simulink model "quadSimplifiedModel"  (R2018b)
settings: Solver=FixedStepAuto  StartTime=0.0  StopTime=tfinal  FixedStep=dt  RelTol=1e-3
values from neighbouring files (symbols this model uses):
  dt = 0.005    [quadSimRunMain.m]    (also in runquadXModel.m)
  Gain = [1 0, 0 0,0 0, 0 0;     0 1, 0 0, 0 0, 0 0;     0 0, param.dt 0, 0 0, 0 0;     0 0, 0 param.dt, 0 0, 0 0;     0 0, 0 0, param.dt^2/2 0, 0 0;     0 0, 0 0, 0 param.dt^2/2, 0 0;     0 0, 0 0, 0 0, 1 0;     0 0, 0 0, 0 0, 0 1]    [quadSimRunMain.m]
  Kdphi = 0.0478*1    (= 0.0478)    [quadSimRunMain.m]
  Kdpsi = 0.067644*1    (= 0.067644)    [quadSimRunMain.m]
  Kdtheta = 0.0478*1    (= 0.0478)    [quadSimRunMain.m]
  Kdx = 15    [quadSimRunMain.m]
  Kdy = 15    [quadSimRunMain.m]
  Kdz = 5.5    [quadSimRunMain.m]
  Kiphi = 0.0098*0    (= 0)    [quadSimRunMain.m]
  Kipsi = 0.045028*.0    (= 0)    [quadSimRunMain.m]
  Kitheta = 0.0098*0    (= 0)    [quadSimRunMain.m]
  Kix = 1    [quadSimRunMain.m]
  Kiy = 1    [quadSimRunMain.m]
  Kiz = 1.5    [quadSimRunMain.m]
  Kpphi = 0.0439*1    (= 0.0439)    [quadSimRunMain.m]
  Kppsi = 0.11038*1    (= 0.11038)    [quadSimRunMain.m]
  Kptheta = 0.0439*1    (= 0.0439)    [quadSimRunMain.m]
  Kpx = 5    [quadSimRunMain.m]
  Kpy = 5    [quadSimRunMain.m]
  Kpz = 3.5    [quadSimRunMain.m]
  Nphi = 1/Tfphi    (= 162.638649449)    [quadSimRunMain.m]
  Npsi = 1/Tfpsi    (= 159.182438993)    [quadSimRunMain.m]
  Ntheta = 1/Tftheta    (= 162.638649449)    [quadSimRunMain.m]
  Nx = 1/0.002099    (= 476.417341591)    [quadSimRunMain.m]
  Ny = 1/0.002099    (= 476.417341591)    [quadSimRunMain.m]
  Nz = 1/0.002099    (= 476.417341591)    [quadSimRunMain.m]
  pathSelect = 1    [quadSimRunMain.m]
  Uphisat = 100*param.m*param.g(3)*0.5    [quadSimRunMain.m]
  Upsisat = 100*param.m*param.g(3)*0.1    [quadSimRunMain.m]
  Uthetasat = 100*param.m*param.g(3)*0.5    [quadSimRunMain.m]
  Uzsat = 100*3*param.m*param.g(3)    [quadSimRunMain.m]
undefined symbols (not defined in the file or in its folder): sigbuilder_block, sigeul, sigpos
libraries: simulink x12
settings Model: Creator=duho46  LastModifiedBy=duho46

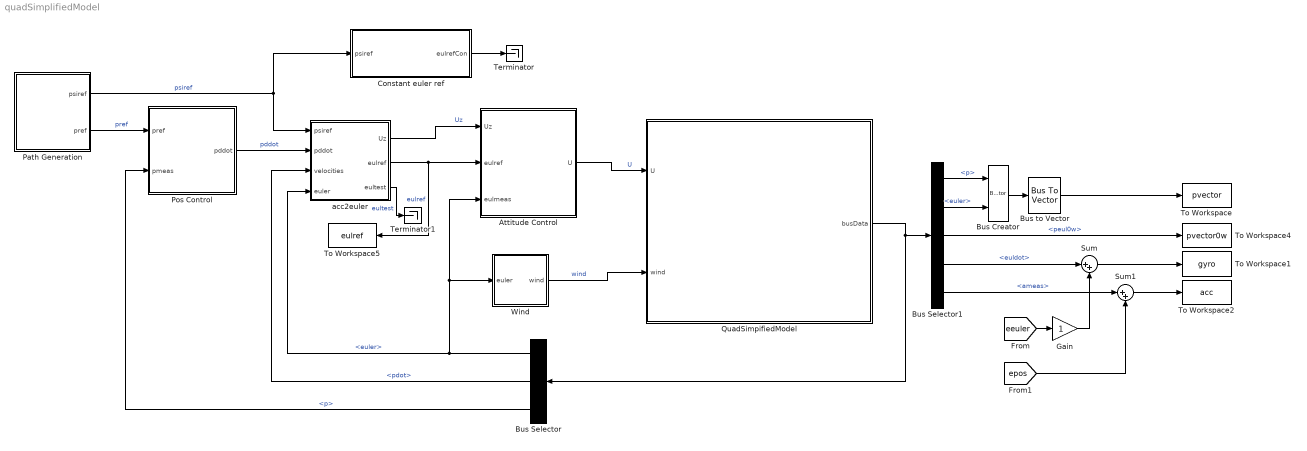
== system quadSimplifiedModel ==
  Attitude Control : Subsystem
      mask Display: image('C:\Users\duho46\Pictures\angles.png');
  Bus Creator : BusCreator  Inputs=2
  Bus Selector : BusSelector  OutputSignals=euler,pdot,p
  Bus Selector1 : BusSelector  OutputSignals=p,euler,peul0w,euldot,ameas
  Bus to Vector : BusToVector
  "Constant euler ref " : Subsystem
  Gain : Gain
  Path Generation : Subsystem
      mask Display: image('C:\Users\duho46\Pictures\96643.png');
  Pos Control : Subsystem
      mask Display: image('C:\Users\duho46\Pictures\control.png');
  QuadSimpifiedModel : Subsystem
      mask Display: image('C:\Users\duho46\Pictures\DJI Mavic Pro.jpg');
  Sum : Sum  Inputs=|++
  Sum1 : Sum  Inputs=|++
  Terminator : Terminator
  Terminator1 : Terminator
  To Workspace : ToWorkspace  VariableName=pvector  SampleTime=-1
  To Workspace1 : ToWorkspace  VariableName=gyro  SampleTime=-1
  To Workspace2 : ToWorkspace  VariableName=acc  SampleTime=-1
  To Workspace4 : ToWorkspace  VariableName=pvector0w  SampleTime=-1
  To Workspace5 : ToWorkspace  VariableName=eulref  SampleTime=-1
  Wind : Subsystem
      mask Display: image('C:\Users\duho46\Pictures\wind.png');
  acc2euler : MATLAB Function  TreatAsAtomicUnit=on
  wires:
  Path Generation/2(pref) -> Pos Control/1(pref)  "pref"
  Pos Control/1(pddot) -> acc2euler/2(pddot)  "pddot"
  acc2euler/1(Uz) -> Attitude Control/1(Uz)  "Uz"
  acc2euler/2(eulref) -> To Workspace5/1, Attitude Control/2(eulref)  "eulref"
  Attitude Control/1(U) -> QuadSimpifiedModel/1(U)  "U"
  Wind/1(wind) -> QuadSimpifiedModel/2(wind)  "wind"
  QuadSimpifiedModel/1(busData) -> Bus Selector/1, Bus Selector1/1
  Bus Selector/1 -> acc2euler/4(euler), Wind/1(euler), Attitude Control/3(eulmeas)  "<euler>"
  Bus Selector/2 -> acc2euler/3(velocities)  "<pdot>"
  Bus Selector/3 -> Pos Control/2(pmeas)  "<p>"
  Bus Selector1/3 -> To Workspace4/1  "<peul0w>"
  Bus to Vector/1 -> To Workspace/1
  Bus Selector1/1 -> Bus Creator/1  "<p>"
  Bus Selector1/2 -> Bus Creator/2  "<euler>"
  Bus Creator/1 -> Bus to Vector/1
  Bus Selector1/4 -> Sum/1  "<euldot>"
  Sum/1 -> To Workspace1/1
  Bus Selector1/5 -> Sum1/1  "<ameas>"
  Sum1/1 -> To Workspace2/1
  [eeuler] -> Gain/1
  [epos] -> Sum1/2
  Gain/1 -> Sum/2
  Path Generation/1(psiref) -> "Constant euler ref "/1(psiref), acc2euler/1(psiref)  "psiref"
  "Constant euler ref "/1(eulrefCon) -> Terminator/1
  acc2euler/3(eultest) -> Terminator1/1  "eultest"

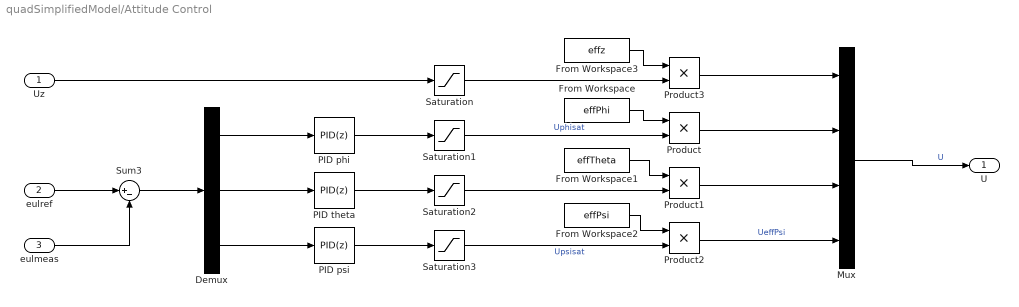
== system quadSimplifiedModel/Attitude Control ==
  Uz : Inport
  eulref : Inport  Port=2
  eulmeas : Inport  Port=3
  Demux : Demux  Outputs=3
  From Workspace : FromWorkspace  VariableName=effPhi  SampleTime=0
  From Workspace1 : FromWorkspace  VariableName=effTheta  SampleTime=0
  From Workspace2 : FromWorkspace  VariableName=effPsi  SampleTime=0
  From Workspace3 : FromWorkspace  VariableName=effz  SampleTime=0
  Mux : Mux
  PID phi : simulink/Continuous/PID Controller  Controller=PID  Form=Parallel  TimeDomain=Discrete-time  SampleTime=-1  IntegratorMethod=Forward Euler  FilterMethod=Forward Euler  ControllerParametersSource=internal  P=Kpphi  I=Kiphi  D=Kdphi  UseFilter=off  N=Nphi  TunerSelectOption=Transfer Function Based (PID Tuner App)  InitialConditionSource=internal  InitialConditionForIntegrator=0  InitialConditionForFilter=0  DifferentiatorICPrevScaledInput=0  ExternalReset=none  TrackingMode=off  Kt=1  LimitOutput=off  UpperSaturationLimit=inf  LowerSaturationLimit=-inf  LinearizeAsGain=on  AntiWindupMode=none  Kb=1  POutMin=[]  POutMax=[]  IOutMin=[]  IOutMax=[]  DOutMin=[]  DOutMax=[]  NOutMin=[]  NOutMax=[]  SumOutMin=[]  SumOutMax=[]  SaturationOutMin=[]  SaturationOutMax=[]  PParamMin=[]  PParamMax=[]  IParamMin=[]  IParamMax=[]  DParamMin=[]  DParamMax=[]  NParamMin=[]  NParamMax=[]  KbParamMin=[]  KbParamMax=[]  KtParamMin=[]  KtParamMax=[]  KbOutMin=[]  KbOutMax=[]  KtOutMin=[]  KtOutMax=[]  IntegratorOutMin=[]  IntegratorOutMax=[]  FilterOutMin=[]  FilterOutMax=[]  SumI1OutMin=[]  SumI1OutMax=[]  SumI2OutMin=[]  SumI2OutMax=[]  SumI3OutMin=[]  SumI3OutMax=[]  SumI4OutMin=[]  SumI4OutMax=[]  SumDOutMin=[]  SumDOutMax=[]  DifferentiatorOutMin=[]  DifferentiatorOutMax=[]  FilterDiffOutCoefMin=[]  FilterDiffOutCoefMax=[]  ReciprocalOutMin=[]  ReciprocalOutMax=[]  SumDenOutMin=[]  SumDenOutMax=[]  SumNumOutMin=[]  SumNumOutMax=[]  DivideOutMin=[]  DivideOutMax=[]  IntegratorContinuousStateAttributes=''  IntegratorStateMustResolveToSignalObject=off  IntegratorRTWStateStorageClass=Auto  FilterContinuousStateAttributes=''  FilterStateMustResolveToSignalObject=off  FilterRTWStateStorageClass=Auto  ParallelPVariant=InternalParameters  IdealPVariant=Disabled  IVariant=InternalParameters  DVariant=InternalParameters  IntegratorVariant=Discrete  SatVariant=Disabled  AWVariant=Passthrough  PCopyVariant=Disabled  TRVariant=Disabled  FdbkBlocksVariant=Forward  IdealPFdbkVariant=Disabled  SatFdbkVariant=Disabled  DerivativeFilterVariant=Differentiator  NVariant=Passthrough  NCopyVariant=Disabled_SignalSpec  FilterICVariant=InternalICsDifferentiator  IntegratorICVariant=InternalICs  ExternalResetVariant=Disabled  TRSumVariant=Passthrough  SumFdbkVariant=Disabled  SumVariant=Sum_PID
  PID psi : simulink/Continuous/PID Controller  Controller=PID  Form=Parallel  TimeDomain=Discrete-time  SampleTime=-1  IntegratorMethod=Forward Euler  FilterMethod=Forward Euler  ControllerParametersSource=internal  P=Kppsi  I=Kipsi  D=Kdpsi  UseFilter=off  N=Npsi  TunerSelectOption=Transfer Function Based (PID Tuner App)  InitialConditionSource=internal  InitialConditionForIntegrator=0  InitialConditionForFilter=0  DifferentiatorICPrevScaledInput=0  ExternalReset=none  TrackingMode=off  Kt=1  LimitOutput=off  UpperSaturationLimit=inf  LowerSaturationLimit=-inf  LinearizeAsGain=on  AntiWindupMode=none  Kb=1  POutMin=[]  POutMax=[]  IOutMin=[]  IOutMax=[]  DOutMin=[]  DOutMax=[]  NOutMin=[]  NOutMax=[]  SumOutMin=[]  SumOutMax=[]  SaturationOutMin=[]  SaturationOutMax=[]  PParamMin=[]  PParamMax=[]  IParamMin=[]  IParamMax=[]  DParamMin=[]  DParamMax=[]  NParamMin=[]  NParamMax=[]  KbParamMin=[]  KbParamMax=[]  KtParamMin=[]  KtParamMax=[]  KbOutMin=[]  KbOutMax=[]  KtOutMin=[]  KtOutMax=[]  IntegratorOutMin=[]  IntegratorOutMax=[]  FilterOutMin=[]  FilterOutMax=[]  SumI1OutMin=[]  SumI1OutMax=[]  SumI2OutMin=[]  SumI2OutMax=[]  SumI3OutMin=[]  SumI3OutMax=[]  SumI4OutMin=[]  SumI4OutMax=[]  SumDOutMin=[]  SumDOutMax=[]  DifferentiatorOutMin=[]  DifferentiatorOutMax=[]  FilterDiffOutCoefMin=[]  FilterDiffOutCoefMax=[]  ReciprocalOutMin=[]  ReciprocalOutMax=[]  SumDenOutMin=[]  SumDenOutMax=[]  SumNumOutMin=[]  SumNumOutMax=[]  DivideOutMin=[]  DivideOutMax=[]  IntegratorContinuousStateAttributes=''  IntegratorStateMustResolveToSignalObject=off  IntegratorRTWStateStorageClass=Auto  FilterContinuousStateAttributes=''  FilterStateMustResolveToSignalObject=off  FilterRTWStateStorageClass=Auto  ParallelPVariant=InternalParameters  IdealPVariant=Disabled  IVariant=InternalParameters  DVariant=InternalParameters  IntegratorVariant=Discrete  SatVariant=Disabled  AWVariant=Passthrough  PCopyVariant=Disabled  TRVariant=Disabled  FdbkBlocksVariant=Forward  IdealPFdbkVariant=Disabled  SatFdbkVariant=Disabled  DerivativeFilterVariant=Differentiator  NVariant=Passthrough  NCopyVariant=Disabled_SignalSpec  FilterICVariant=InternalICsDifferentiator  IntegratorICVariant=InternalICs  ExternalResetVariant=Disabled  TRSumVariant=Passthrough  SumFdbkVariant=Disabled  SumVariant=Sum_PID
  PID theta : simulink/Continuous/PID Controller  Controller=PID  Form=Parallel  TimeDomain=Discrete-time  SampleTime=-1  IntegratorMethod=Forward Euler  FilterMethod=Forward Euler  ControllerParametersSource=internal  P=Kptheta  I=Kitheta  D=Kdtheta  UseFilter=off  N=Ntheta  TunerSelectOption=Transfer Function Based (PID Tuner App)  InitialConditionSource=internal  InitialConditionForIntegrator=0  InitialConditionForFilter=0  DifferentiatorICPrevScaledInput=0  ExternalReset=none  TrackingMode=off  Kt=1  LimitOutput=off  UpperSaturationLimit=inf  LowerSaturationLimit=-inf  LinearizeAsGain=on  AntiWindupMode=none  Kb=1  POutMin=[]  POutMax=[]  IOutMin=[]  IOutMax=[]  DOutMin=[]  DOutMax=[]  NOutMin=[]  NOutMax=[]  SumOutMin=[]  SumOutMax=[]  SaturationOutMin=[]  SaturationOutMax=[]  PParamMin=[]  PParamMax=[]  IParamMin=[]  IParamMax=[]  DParamMin=[]  DParamMax=[]  NParamMin=[]  NParamMax=[]  KbParamMin=[]  KbParamMax=[]  KtParamMin=[]  KtParamMax=[]  KbOutMin=[]  KbOutMax=[]  KtOutMin=[]  KtOutMax=[]  IntegratorOutMin=[]  IntegratorOutMax=[]  FilterOutMin=[]  FilterOutMax=[]  SumI1OutMin=[]  SumI1OutMax=[]  SumI2OutMin=[]  SumI2OutMax=[]  SumI3OutMin=[]  SumI3OutMax=[]  SumI4OutMin=[]  SumI4OutMax=[]  SumDOutMin=[]  SumDOutMax=[]  DifferentiatorOutMin=[]  DifferentiatorOutMax=[]  FilterDiffOutCoefMin=[]  FilterDiffOutCoefMax=[]  ReciprocalOutMin=[]  ReciprocalOutMax=[]  SumDenOutMin=[]  SumDenOutMax=[]  SumNumOutMin=[]  SumNumOutMax=[]  DivideOutMin=[]  DivideOutMax=[]  IntegratorContinuousStateAttributes=''  IntegratorStateMustResolveToSignalObject=off  IntegratorRTWStateStorageClass=Auto  FilterContinuousStateAttributes=''  FilterStateMustResolveToSignalObject=off  FilterRTWStateStorageClass=Auto  ParallelPVariant=InternalParameters  IdealPVariant=Disabled  IVariant=InternalParameters  DVariant=InternalParameters  IntegratorVariant=Discrete  SatVariant=Disabled  AWVariant=Passthrough  PCopyVariant=Disabled  TRVariant=Disabled  FdbkBlocksVariant=Forward  IdealPFdbkVariant=Disabled  SatFdbkVariant=Disabled  DerivativeFilterVariant=Differentiator  NVariant=Passthrough  NCopyVariant=Disabled_SignalSpec  FilterICVariant=InternalICsDifferentiator  IntegratorICVariant=InternalICs  ExternalResetVariant=Disabled  TRSumVariant=Passthrough  SumFdbkVariant=Disabled  SumVariant=Sum_PID
  Product{,1..3} (4 alike) : Product
  Saturation : Saturate  UpperLimit=Uzsat  LowerLimit=-Uzsat
  Saturation1 : Saturate  UpperLimit=Uphisat  LowerLimit=-Uphisat
  Saturation2 : Saturate  UpperLimit=Uthetasat  LowerLimit=-Uthetasat
  Saturation3 : Saturate  UpperLimit=Upsisat  LowerLimit=-Upsisat
  Sum3 : Sum  Inputs=|+-
  U : Outport
  wires:
  PID phi/1 -> Saturation1/1
  Mux/1 -> U/1  "U"
  Demux/3 -> PID psi/1
  PID theta/1 -> Saturation2/1
  PID psi/1 -> Saturation3/1
  Demux/2 -> PID theta/1
  Uz/1 -> Saturation/1
  Sum3/1 -> Demux/1
  eulref/1 -> Sum3/1
  eulmeas/1 -> Sum3/2
  Demux/1 -> PID phi/1
  Saturation1/1 -> Product/2  "Uphisat"
  From Workspace/1 -> Product/1
  Product/1 -> Mux/2
  Product1/1 -> Mux/3
  Product2/1 -> Mux/4  "UeffPsi"
  Saturation3/1 -> Product2/2  "Upsisat"
  Saturation2/1 -> Product1/2
  From Workspace1/1 -> Product1/1
  From Workspace2/1 -> Product2/1
  Product3/1 -> Mux/1
  Saturation/1 -> Product3/2
  From Workspace3/1 -> Product3/1

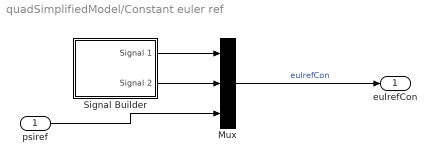
== system quadSimplifiedModel/Constant euler ref  ==
  psiref : Inport
  Mux : Mux  Inputs=3
  Signal Builder : Subsystem  Tag=STV Subsys  LoadFcn=sigbuilder_block('load');  StartFcn=sigbuilder_block('start');  StopFcn=sigbuilder_block('stop');  ClipboardFcn=sigbuilder_block('clipboard');  mask(Sigbuilder block){tuvar=[0:10]}
      mask help: Simulink:masks:SigbuilderBlock_MD
      mask init:
      | if ~strcmp(get_param(bdroot(gcbh),'SimulationStatus'),'stopped') tuvar = sigbuilder_block('maskInit'); end
      settings: CopyFcn=sigbuilder_block('copy');  DeleteFcn=sigbuilder_block('delete');  ModelCloseFcn=sigbuilder_block('modelClose');  PreSaveFcn=sigbuilder_block('preSave');  PauseFcn=sigbuilder_block('pause');  ContinueFcn=sigbuilder_block('continue');  NameChangeFcn=sigbuilder_block('namechange');  OpenFcn=sigbuilder_block('open',[1692 200.25 550.5 399.75 ]);  CloseFcn=sigbuilder_block('close');
      mask Display: plot(0, 0, 100, 100,[2, 2, 32, 32, 2], [68, 8, 8, 68, 68],[32, 2], [38, 38], [32, 19, 2],[53, 60, 44], [32, 17, 17, 2],[16, 16, 31, 31]);txt = getActiveGroup(gcbh);text(2, 100, txt,'verticalAlignment', 'top');
  eulrefCon : Outport
  wires:
  Signal Builder/1(Signal 1) -> Mux/1
  psiref/1 -> Mux/3
  Mux/1 -> eulrefCon/1  "eulrefCon"
  Signal Builder/2(Signal 2) -> Mux/2

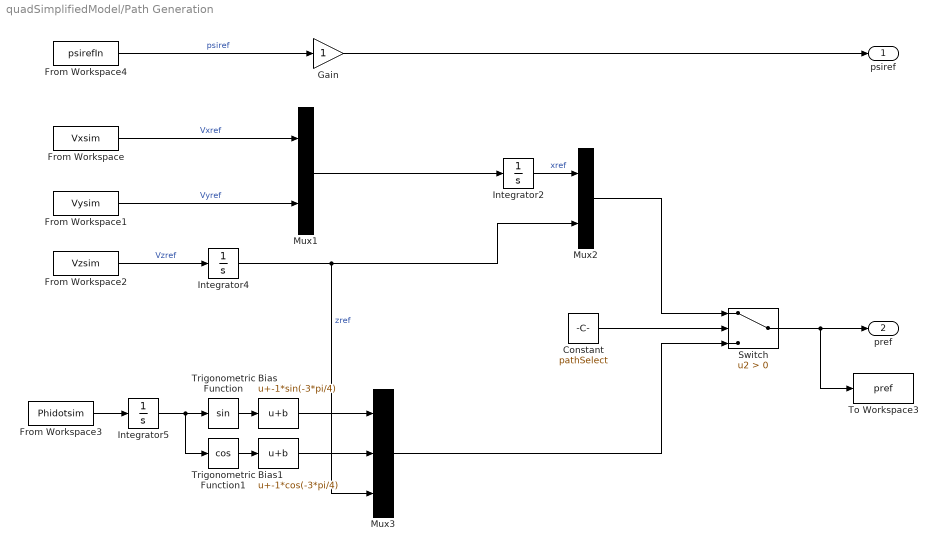
== system quadSimplifiedModel/Path Generation ==
  Bias : Bias  Bias=-1*sin(-3*pi/4)
  Bias1 : Bias  Bias=-1*cos(-3*pi/4)
  Constant : Constant  Value=pathSelect
  From Workspace : FromWorkspace  VariableName=Vxsim  SampleTime=0
  From Workspace1 : FromWorkspace  VariableName=Vysim  SampleTime=0
  From Workspace2 : FromWorkspace  VariableName=Vzsim  SampleTime=0
  From Workspace3 : FromWorkspace  VariableName=Phidotsim  SampleTime=0
  From Workspace4 : FromWorkspace  VariableName=psirefIn  SampleTime=0
  Gain : Gain
  Integrator2 : Integrator
  Integrator4 : Integrator
  Integrator5 : Integrator  InitialCondition=-3*pi/4
  Mux1 : Mux  Inputs=2
  Mux2 : Mux  Inputs=2
  Mux3 : Mux  Inputs=3
  Switch : Switch  Criteria=u2 > Threshold
  To Workspace3 : ToWorkspace  VariableName=pref  SampleTime=-1
  Trigonometric Function : Trigonometry
  Trigonometric Function1 : Trigonometry  Operator=cos
  psiref : Outport
  pref : Outport  Port=2
  wires:
  Integrator4/1 -> Mux3/3, Mux2/2  "zref"
  From Workspace2/1 -> Integrator4/1  "Vzref"
  Integrator5/1 -> Trigonometric Function1/1, Trigonometric Function/1
  From Workspace3/1 -> Integrator5/1
  Trigonometric Function1/1 -> Bias1/1
  Trigonometric Function/1 -> Bias/1
  Bias/1 -> Mux3/1
  Bias1/1 -> Mux3/2
  From Workspace4/1 -> Gain/1  "psiref"
  Mux1/1 -> Integrator2/1
  Integrator2/1 -> Mux2/1  "xref"
  From Workspace/1 -> Mux1/1  "Vxref"
  From Workspace1/1 -> Mux1/2  "Vyref"
  Gain/1 -> psiref/1
  Switch/1 -> To Workspace3/1, pref/1
  Mux2/1 -> Switch/1
  Mux3/1 -> Switch/3
  Constant/1 -> Switch/2

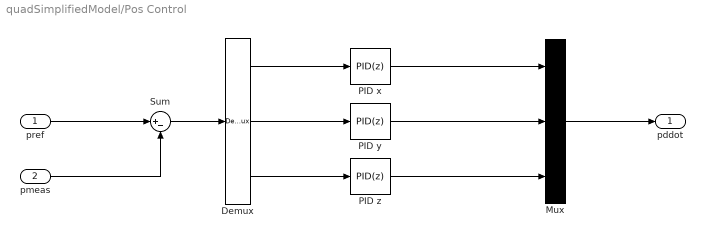
== system quadSimplifiedModel/Pos Control ==
  pref : Inport
  pmeas : Inport  Port=2
  Demux : Demux  Outputs=3
  Mux : Mux  Inputs=3
  PID x : simulink/Continuous/PID Controller  Controller=PID  Form=Parallel  TimeDomain=Discrete-time  SampleTime=-1  IntegratorMethod=Forward Euler  FilterMethod=Forward Euler  ControllerParametersSource=internal  P=Kpx  I=Kix  D=Kdx  UseFilter=off  N=Nx  TunerSelectOption=Transfer Function Based (PID Tuner App)  InitialConditionSource=internal  InitialConditionForIntegrator=0  InitialConditionForFilter=0  DifferentiatorICPrevScaledInput=0  ExternalReset=none  TrackingMode=off  Kt=1  LimitOutput=off  UpperSaturationLimit=inf  LowerSaturationLimit=-inf  LinearizeAsGain=on  AntiWindupMode=none  Kb=1  POutMin=[]  POutMax=[]  IOutMin=[]  IOutMax=[]  DOutMin=[]  DOutMax=[]  NOutMin=[]  NOutMax=[]  SumOutMin=[]  SumOutMax=[]  SaturationOutMin=[]  SaturationOutMax=[]  PParamMin=[]  PParamMax=[]  IParamMin=[]  IParamMax=[]  DParamMin=[]  DParamMax=[]  NParamMin=[]  NParamMax=[]  KbParamMin=[]  KbParamMax=[]  KtParamMin=[]  KtParamMax=[]  KbOutMin=[]  KbOutMax=[]  KtOutMin=[]  KtOutMax=[]  IntegratorOutMin=[]  IntegratorOutMax=[]  FilterOutMin=[]  FilterOutMax=[]  SumI1OutMin=[]  SumI1OutMax=[]  SumI2OutMin=[]  SumI2OutMax=[]  SumI3OutMin=[]  SumI3OutMax=[]  SumI4OutMin=[]  SumI4OutMax=[]  SumDOutMin=[]  SumDOutMax=[]  DifferentiatorOutMin=[]  DifferentiatorOutMax=[]  FilterDiffOutCoefMin=[]  FilterDiffOutCoefMax=[]  ReciprocalOutMin=[]  ReciprocalOutMax=[]  SumDenOutMin=[]  SumDenOutMax=[]  SumNumOutMin=[]  SumNumOutMax=[]  DivideOutMin=[]  DivideOutMax=[]  IntegratorContinuousStateAttributes=''  IntegratorStateMustResolveToSignalObject=off  IntegratorRTWStateStorageClass=Auto  FilterContinuousStateAttributes=''  FilterStateMustResolveToSignalObject=off  FilterRTWStateStorageClass=Auto  ParallelPVariant=InternalParameters  IdealPVariant=Disabled  IVariant=InternalParameters  DVariant=InternalParameters  IntegratorVariant=Discrete  SatVariant=Disabled  AWVariant=Passthrough  PCopyVariant=Disabled  TRVariant=Disabled  FdbkBlocksVariant=Forward  IdealPFdbkVariant=Disabled  SatFdbkVariant=Disabled  DerivativeFilterVariant=Differentiator  NVariant=Passthrough  NCopyVariant=Disabled_SignalSpec  FilterICVariant=InternalICsDifferentiator  IntegratorICVariant=InternalICs  ExternalResetVariant=Disabled  TRSumVariant=Passthrough  SumFdbkVariant=Disabled  SumVariant=Sum_PID
  PID y : simulink/Continuous/PID Controller  Controller=PID  Form=Parallel  TimeDomain=Discrete-time  SampleTime=-1  IntegratorMethod=Forward Euler  FilterMethod=Forward Euler  ControllerParametersSource=internal  P=Kpy  I=Kiy  D=Kdy  UseFilter=off  N=Ny  TunerSelectOption=Transfer Function Based (PID Tuner App)  InitialConditionSource=internal  InitialConditionForIntegrator=0  InitialConditionForFilter=0  DifferentiatorICPrevScaledInput=0  ExternalReset=none  TrackingMode=off  Kt=1  LimitOutput=off  UpperSaturationLimit=inf  LowerSaturationLimit=-inf  LinearizeAsGain=on  AntiWindupMode=none  Kb=1  POutMin=[]  POutMax=[]  IOutMin=[]  IOutMax=[]  DOutMin=[]  DOutMax=[]  NOutMin=[]  NOutMax=[]  SumOutMin=[]  SumOutMax=[]  SaturationOutMin=[]  SaturationOutMax=[]  PParamMin=[]  PParamMax=[]  IParamMin=[]  IParamMax=[]  DParamMin=[]  DParamMax=[]  NParamMin=[]  NParamMax=[]  KbParamMin=[]  KbParamMax=[]  KtParamMin=[]  KtParamMax=[]  KbOutMin=[]  KbOutMax=[]  KtOutMin=[]  KtOutMax=[]  IntegratorOutMin=[]  IntegratorOutMax=[]  FilterOutMin=[]  FilterOutMax=[]  SumI1OutMin=[]  SumI1OutMax=[]  SumI2OutMin=[]  SumI2OutMax=[]  SumI3OutMin=[]  SumI3OutMax=[]  SumI4OutMin=[]  SumI4OutMax=[]  SumDOutMin=[]  SumDOutMax=[]  DifferentiatorOutMin=[]  DifferentiatorOutMax=[]  FilterDiffOutCoefMin=[]  FilterDiffOutCoefMax=[]  ReciprocalOutMin=[]  ReciprocalOutMax=[]  SumDenOutMin=[]  SumDenOutMax=[]  SumNumOutMin=[]  SumNumOutMax=[]  DivideOutMin=[]  DivideOutMax=[]  IntegratorContinuousStateAttributes=''  IntegratorStateMustResolveToSignalObject=off  IntegratorRTWStateStorageClass=Auto  FilterContinuousStateAttributes=''  FilterStateMustResolveToSignalObject=off  FilterRTWStateStorageClass=Auto  ParallelPVariant=InternalParameters  IdealPVariant=Disabled  IVariant=InternalParameters  DVariant=InternalParameters  IntegratorVariant=Discrete  SatVariant=Disabled  AWVariant=Passthrough  PCopyVariant=Disabled  TRVariant=Disabled  FdbkBlocksVariant=Forward  IdealPFdbkVariant=Disabled  SatFdbkVariant=Disabled  DerivativeFilterVariant=Differentiator  NVariant=Passthrough  NCopyVariant=Disabled_SignalSpec  FilterICVariant=InternalICsDifferentiator  IntegratorICVariant=InternalICs  ExternalResetVariant=Disabled  TRSumVariant=Passthrough  SumFdbkVariant=Disabled  SumVariant=Sum_PID
  PID z : simulink/Continuous/PID Controller  Controller=PID  Form=Parallel  TimeDomain=Discrete-time  SampleTime=-1  IntegratorMethod=Forward Euler  FilterMethod=Forward Euler  ControllerParametersSource=internal  P=Kpz  I=Kiz  D=Kdz  UseFilter=off  N=Nz  TunerSelectOption=Transfer Function Based (PID Tuner App)  InitialConditionSource=internal  InitialConditionForIntegrator=0  InitialConditionForFilter=0  DifferentiatorICPrevScaledInput=0  ExternalReset=none  TrackingMode=off  Kt=1  LimitOutput=off  UpperSaturationLimit=inf  LowerSaturationLimit=-inf  LinearizeAsGain=on  AntiWindupMode=none  Kb=1  POutMin=[]  POutMax=[]  IOutMin=[]  IOutMax=[]  DOutMin=[]  DOutMax=[]  NOutMin=[]  NOutMax=[]  SumOutMin=[]  SumOutMax=[]  SaturationOutMin=[]  SaturationOutMax=[]  PParamMin=[]  PParamMax=[]  IParamMin=[]  IParamMax=[]  DParamMin=[]  DParamMax=[]  NParamMin=[]  NParamMax=[]  KbParamMin=[]  KbParamMax=[]  KtParamMin=[]  KtParamMax=[]  KbOutMin=[]  KbOutMax=[]  KtOutMin=[]  KtOutMax=[]  IntegratorOutMin=[]  IntegratorOutMax=[]  FilterOutMin=[]  FilterOutMax=[]  SumI1OutMin=[]  SumI1OutMax=[]  SumI2OutMin=[]  SumI2OutMax=[]  SumI3OutMin=[]  SumI3OutMax=[]  SumI4OutMin=[]  SumI4OutMax=[]  SumDOutMin=[]  SumDOutMax=[]  DifferentiatorOutMin=[]  DifferentiatorOutMax=[]  FilterDiffOutCoefMin=[]  FilterDiffOutCoefMax=[]  ReciprocalOutMin=[]  ReciprocalOutMax=[]  SumDenOutMin=[]  SumDenOutMax=[]  SumNumOutMin=[]  SumNumOutMax=[]  DivideOutMin=[]  DivideOutMax=[]  IntegratorContinuousStateAttributes=''  IntegratorStateMustResolveToSignalObject=off  IntegratorRTWStateStorageClass=Auto  FilterContinuousStateAttributes=''  FilterStateMustResolveToSignalObject=off  FilterRTWStateStorageClass=Auto  ParallelPVariant=InternalParameters  IdealPVariant=Disabled  IVariant=InternalParameters  DVariant=InternalParameters  IntegratorVariant=Discrete  SatVariant=Disabled  AWVariant=Passthrough  PCopyVariant=Disabled  TRVariant=Disabled  FdbkBlocksVariant=Forward  IdealPFdbkVariant=Disabled  SatFdbkVariant=Disabled  DerivativeFilterVariant=Differentiator  NVariant=Passthrough  NCopyVariant=Disabled_SignalSpec  FilterICVariant=InternalICsDifferentiator  IntegratorICVariant=InternalICs  ExternalResetVariant=Disabled  TRSumVariant=Passthrough  SumFdbkVariant=Disabled  SumVariant=Sum_PID
  Sum : Sum  Inputs=|+-
  pddot : Outport
  wires:
  Demux/3 -> PID z/1
  PID x/1 -> Mux/1
  PID y/1 -> Mux/2
  PID z/1 -> Mux/3
  Mux/1 -> pddot/1
  pref/1 -> Sum/1
  pmeas/1 -> Sum/2
  Demux/1 -> PID x/1
  Demux/2 -> PID y/1
  Sum/1 -> Demux/1

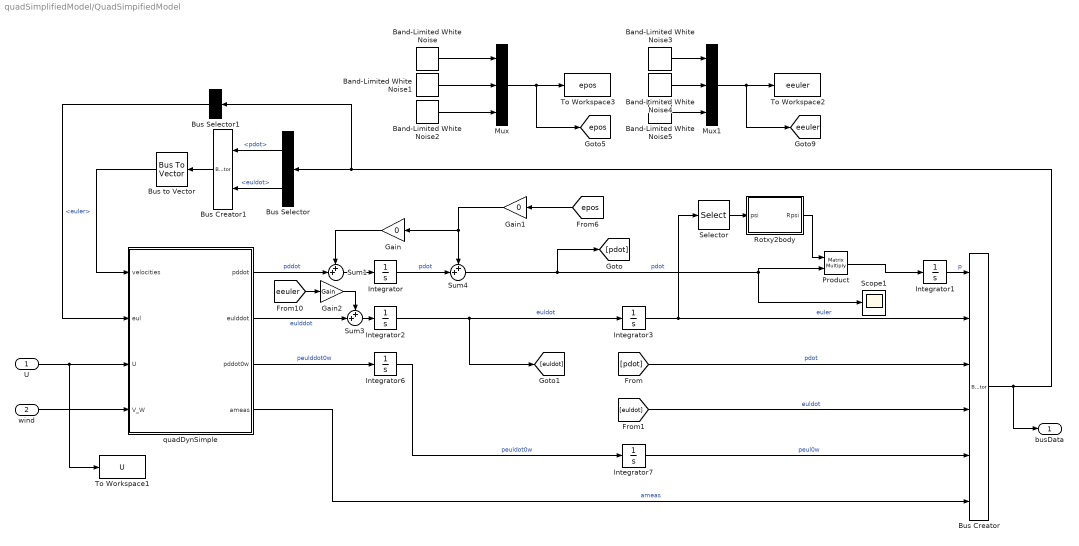
== system quadSimplifiedModel/QuadSimpifiedModel ==
  U : Inport
  wind : Inport  Port=2
  Band-Limited White Noise : simulink/Sources/Band-Limited White Noise  Cov=[sigpos*dt]  Ts=dt  seed=[randi(1e6)]
  Band-Limited White Noise1 : simulink/Sources/Band-Limited White Noise  Cov=[sigpos*dt]  Ts=dt  seed=[randi(1e6)]
  Band-Limited White Noise2 : simulink/Sources/Band-Limited White Noise  Cov=[sigpos*dt]  Ts=dt  seed=[randi(1e6)]
  Band-Limited White Noise3 : simulink/Sources/Band-Limited White Noise  Cov=[sigeul*dt]  Ts=dt  seed=[randi(1e6)]
  Band-Limited White Noise4 : simulink/Sources/Band-Limited White Noise  Cov=[sigeul*dt]  Ts=dt  seed=[randi(1e6)]
  Band-Limited White Noise5 : simulink/Sources/Band-Limited White Noise  Cov=[sigeul*dt]  Ts=dt  seed=[randi(1e6)]
  Bus Creator : BusCreator  Inputs=6
  Bus Creator1 : BusCreator  Inputs=2
  Bus Selector : BusSelector  OutputSignals=pdot,euldot
  Bus Selector1 : BusSelector  OutputSignals=euler
  Bus to Vector : BusToVector
  Gain : Gain  Gain=0
  Gain1 : Gain  Gain=0
  Gain2 : Gain  Gain=Gain
  Integrator : Integrator  InitialCondition=[0 0 0]
  Integrator1 : Integrator  InitialCondition=[0 0 0]
  Integrator2 : Integrator  InitialCondition=[0 0 0]
  Integrator3 : Integrator  InitialCondition=[0 0 0.1]
  Integrator6 : Integrator  InitialCondition=[0 0 0 0 0 0]
  Integrator7 : Integrator  InitialCondition=[0 0 0 0 0 0]
  Mux : Mux  Inputs=3
  Mux1 : Mux  Inputs=3
  Product : Product  Multiplication=Matrix(*)
  Rotxy2body : MATLAB Function  TreatAsAtomicUnit=on
  Scope1 : Scope
  Selector : Selector  InputPortWidth=3  IndexOptions=Index vector (dialog)  Indices=3  OutputSizes=1
  Sum1 : Sum  Inputs=++|
  Sum3 : Sum  Inputs=++|
  Sum4 : Sum  Inputs=++|
  To Workspace1 : ToWorkspace  VariableName=U  SampleTime=-1
  To Workspace2 : ToWorkspace  VariableName=eeuler  SampleTime=-1
  To Workspace3 : ToWorkspace  VariableName=epos  SampleTime=-1
  quadDynSimple : MATLAB Function  TreatAsAtomicUnit=on
  busData : Outport
  tag scope: eeuler=global, epos=global
  wires:
  wind/1 -> quadDynSimple/4(V_W)
  Integrator6/1 -> Integrator7/1  "peuldot0w"
  quadDynSimple/3(pddot0w) -> Integrator6/1  "peulddot0w"
  U/1 -> To Workspace1/1, quadDynSimple/3(U)
  Integrator1/1 -> Bus Creator/1  "p"
  Integrator7/1 -> Bus Creator/5  "peul0w"
  Bus Creator/1 -> busData/1, Bus Selector1/1, Bus Selector/1
  Bus Selector/1 -> Bus Creator1/1  "<pdot>"
  Bus Selector/2 -> Bus Creator1/2  "<euldot>"
  Bus Creator1/1 -> Bus to Vector/1
  Bus to Vector/1 -> quadDynSimple/1(velocities)
  Bus Selector1/1 -> quadDynSimple/2(eul)  "<euler>"
  [pdot] -> Bus Creator/3  "pdot"
  Integrator3/1 -> Selector/1, Bus Creator/2  "euler"
  Mux/1 -> [epos], To Workspace3/1
  Integrator2/1 -> Integrator3/1, [euldot]  "euldot"
  quadDynSimple/1(pddot) -> Sum1/2  "pddot"
  [epos] -> Gain1/1
  Mux1/1 -> To Workspace2/1, [eeuler]
  Sum1/1 -> Integrator/1
  quadDynSimple/2(eulddot) -> Sum3/2  "eulddot"
  Sum3/1 -> Integrator2/1
  [eeuler] -> Gain2/1
  Band-Limited White Noise1/1 -> Mux/2
  Band-Limited White Noise/1 -> Mux/1
  Band-Limited White Noise2/1 -> Mux/3
  Band-Limited White Noise4/1 -> Mux1/2
  Band-Limited White Noise5/1 -> Mux1/3
  Band-Limited White Noise3/1 -> Mux1/1
  Integrator/1 -> Sum4/2  "pdot"
  Sum4/1 -> [pdot], Scope1/1, Product/2  "pdot"
  Gain/1 -> Sum1/1
  Gain1/1 -> Gain/1, Sum4/1
  [euldot] -> Bus Creator/4  "euldot"
  quadDynSimple/4(ameas) -> Bus Creator/6  "ameas"
  Gain2/1 -> Sum3/1
  Selector/1 -> Rotxy2body/1(psi)
  Rotxy2body/1(Rpsi) -> Product/1
  Product/1 -> Integrator1/1

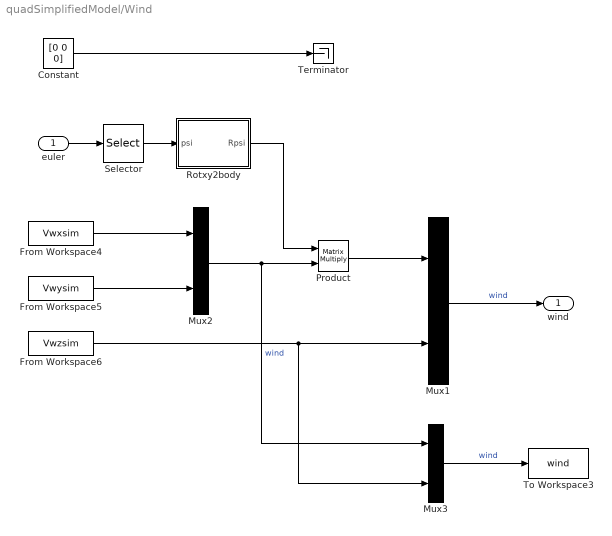
== system quadSimplifiedModel/Wind ==
  euler : Inport
  Constant : Constant  Value=[0 0 0]
  From Workspace4 : FromWorkspace  VariableName=Vwxsim  SampleTime=0
  From Workspace5 : FromWorkspace  VariableName=Vwysim  SampleTime=0
  From Workspace6 : FromWorkspace  VariableName=Vwzsim  SampleTime=0
  Mux1 : Mux  Inputs=2
  Mux2 : Mux  Inputs=2
  Mux3 : Mux  Inputs=2
  Product : Product  Multiplication=Matrix(*)
  Rotxy2body : MATLAB Function  TreatAsAtomicUnit=on
  Selector : Selector  InputPortWidth=3  IndexOptions=Index vector (dialog)  Indices=3  OutputSizes=1
  Terminator : Terminator
  To Workspace3 : ToWorkspace  VariableName=wind  SampleTime=-1
  wind : Outport
  wires:
  Mux1/1 -> wind/1  "wind"
  Constant/1 -> Terminator/1
  euler/1 -> Selector/1
  Selector/1 -> Rotxy2body/1(psi)
  From Workspace6/1 -> Mux3/2, Mux1/2
  From Workspace4/1 -> Mux2/1
  From Workspace5/1 -> Mux2/2
  Mux2/1 -> Mux3/1, Product/2  "wind"
  Rotxy2body/1(Rpsi) -> Product/1
  Product/1 -> Mux1/1
  Mux3/1 -> To Workspace3/1  "wind"

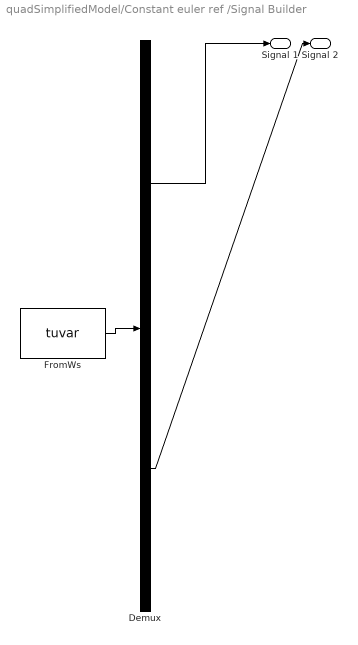
== system quadSimplifiedModel/Constant euler ref /Signal Builder ==
  Demux : Demux  Tag=STV Demux  Outputs=2
  FromWs : FromWorkspace  Tag=STV FromWs  VariableName=tuvar  SampleTime=0
      SigBuilderData=|
      | common.afterFinalStr = 'Extrapolate'
      | common.sampleTime = 0
      | dataSet.timeRange = [0 120]
      | dataSet.name = 'Group 1'
      | sbobj.Groups.Name = 'Group 1'
      | sbobj.Groups.Signals(1).Name = 'Signal 1'
      | sbobj.Groups.Signals(1).XData = [0 20 20 100 100 120]
      | sbobj.Groups.Signals(1).YData = [0 0 0.1 0.1 0 0]
      | sbobj.Groups.Signals(2).Name = 'Signal 2'
      | sbobj.Groups.Signals(2).XData = [0 20 20 100 100 120]
      | sbobj.Groups.Signals(2).YData = [0 0 0.1 0.1 0 0]
      | sbobj.Groups.TimeRange = [0 120]
  Signal 1 : Outport  Tag=STV Outport
  Signal 2 : Outport  Tag=STV Outport  Port=2
  wires:
  Demux/1 -> Signal 1/1
  FromWs/1 -> Demux/1
  Demux/2 -> Signal 2/1

== matlab function quadSimplifiedModel/acc2euler ==
  data: psiref input; pddot input; Uz output; velocities input; eulref output; euler input; eultest output
function [Uz, eulref,eultest] = acce2forces(psiref,pddot,velocities,euler)

param.m = 0.5;
param.g = [0 0 9.81]';
param.cd = 0.32;
param.cf = 1e-4;
param.L = 0.5;
param.ct = 1e-5;
param.Jx = 0.002;
param.Jy = 0.002;
param.Jz = 0.003;
param.lambda1 = 0.36;
param.lambda2 = 0.6;
param.alpha1 = 0.002;
param.alpha2 = 0.005;

% pddot = 1/param.m*([0 0 U(1)]' - param.lambda1*[pdot(1)+u_w; pdot(2)+v_w; pdot(3)+w_w] + ...
%     param.g(3)*[euler(2); -euler(1); 0]);

u = velocities(1);v = velocities(2);w = velocities(3);
uddot = pddot(1); 
vddot = pddot(2); 
wddot = pddot(3);

% Rpsi = [cos(psiref) sin(psiref) 0;-sin(psiref) cos(psiref) 0; 0 0 1];
% pddotRot = Rpsi*pddot;

thetatest = (uddot*cos(psiref)+vddot*sin(psiref) + 0*param.lambda1/param.m*u)/param.g(3);
phitest = (uddot*sin(psiref)-vddot*cos(psiref) + 0*param.lambda1/param.m*v)/param.g(3);

theta = (uddot + 0*param.lambda1/param.m*u)/param.g(3); %uddot
phi = -(vddot + 0*param.lambda1/param.m*v)/param.g(3); % vddot
Uz = param.m*(wddot + param.g(3)) + 0*param.lambda1*w; %wddot
eulref = [phitest; thetatest; psiref];
eultest = [phi;theta;psiref];

== matlab function quadSimplifiedModel/QuadSimpifiedModel/quadDynSimple ==
  data: velocities input; eul input; U input; V_W input; pddot output; eulddot output; pddot0w output; ameas output
function [pddot, eulddot, pddot0w, ameas] = quadDynSimple(velocities,eul,U,V_W)
%quadDynSimple Simplified translation and rotation of quadcopter
%   euler: the Euler angles of quadcopter
%   U: The control signal around trim condition: U_z tau_phi tau_theta
%   tau_psi
%   V_W: wind velocity: u_w v_w w_w

param.m = 0.5;
param.g = [0 0 9.81]';
param.cd = 0.32;
param.cf = 1e-4;
param.L = 0.5;
param.ct = 1e-5;
param.Jx = 0.002;
param.Jy = 0.002;
param.Jz = 0.003;
param.lambda1 = 0.36;
param.lambda2 = 0.6;
param.alpha1 = 0.002;
param.alpha2 = 0.005;

param.alphaphi = 0.002;

pdot = velocities(1:3);
eulerdot = velocities(4:6);
u_w = V_W(1);v_w = V_W(2);w_w = V_W(3);
Seuldot = [0 -eulerdot(3) eulerdot(2);...
    eulerdot(3) 0 -eulerdot(1);...
    -eulerdot(2) eulerdot(1) 0];

% Compute the translational and rotational acceleartions with wind effect
ameas= 1/param.m*([0 0 U(1)]' - param.lambda1*[pdot(1)+u_w; pdot(2)+v_w;...
    param.lambda2/param.lambda1*(pdot(3)+w_w)]);
pddot = ameas + param.g(3)*[eul(2); -eul(1); -1] - Seuldot*pdot;
ameas = -ameas; % Have a form of a - g
eulddot = [U(2)/param.Jx ; U(3)/param.Jy - param.alphaphi*u_w/param.Jy; U(4)/param.Jz] -...
    [param.alpha1*eulerdot(1)/param.Jx; param.alpha1*eulerdot(2)/param.Jy;...
    param.alpha2*eulerdot(3)/param.Jz];

% Compute the translational and rotational acceleartions without wind effect
pddotn = 1/param.m*([0 0 U(1)]' - param.lambda1*[pdot(1)+0; pdot(2)+0;...
    param.lambda2/param.lambda1*(pdot(3)+0)]) + ...
    param.g(3)*[eul(2); -eul(1); -1];
pddot0w = [pddotn;eulddot];
end

== matlab function quadSimplifiedModel/QuadSimpifiedModel/Rotxy2body ==
  data: psi input; Rpsi output
function Rpsi = rotPsi(psi)
Rpsi = [cos(psi) -sin(psi) 0;sin(psi) cos(psi) 0;0 0 1];

== matlab function quadSimplifiedModel/Wind/Rotxy2body ==
  data: psi input; Rpsi output
function Rpsi = rotPsi(psi)
Rpsi = [cos(psi) sin(psi);-sin(psi) cos(psi)];
